simulink model "GMCLIB_Park_BAM_F32"  (Simulink 8.3)
settings: Solver=ode45  StartTime=0.0  StopTime=10.0  RelTol=1e-3
settings Model: Creator=RE004C  LastModifiedBy=B17364
settings OptimizationCC: ExpressionDepthLimit=2147483647
settings DebuggingCC: FcnCallInpInsideContextMsg=UseLocalSettings  StrictBusMsg=Warning
settings HardwareCC: ProdLargestAtomicInteger=Long  ProdLargestAtomicFloat=Double  ProdIntDivRoundTo=Zero  ProdEndianess=BigEndian  ProdHWDeviceType=Freescale->32-bit PowerPC

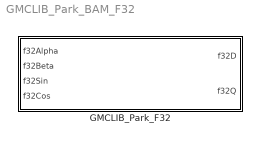
== system GMCLIB_Park_BAM_F32 ==
  GMCLIB_Park_F32 : Subsystem  mask(GMCLIB_Park_F32){}
      mask help: Bit accurate model of Park transformation 2ph stationary -> 2ph rotational.
      mask init:
      | pos = get_param(gcb, 'Position');width = pos(3) - pos(1); height = pos(4) - pos(2);tX=width/2;tY=height*0.9;
      mask Display: color('black');port_label('input',1,'f32Alpha');port_label('input',2,'f32Beta');port_label('input',3,'f32Sin');port_label('input',4,'f32Cos');port_label('output',1,'f32D');port_label('output',2,'f32Q');color('black');disp('GMCLIB_Park_F32');color('blue');text(tX,tY, 'BAM', 'horizontalAlignment', 'center');

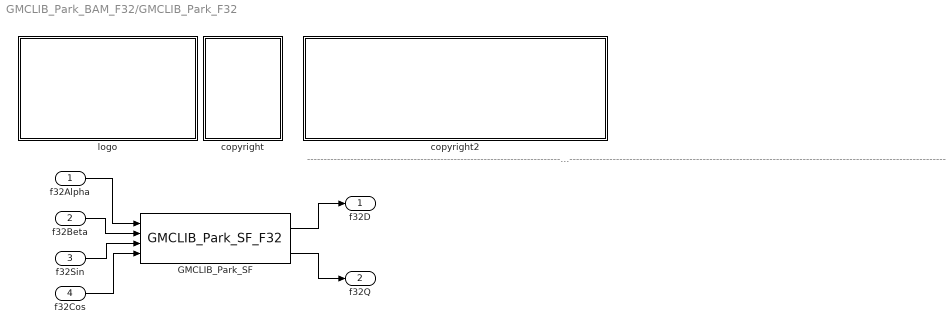
== system GMCLIB_Park_BAM_F32/GMCLIB_Park_F32 ==
  note: ---------------------------------------------------------------------------------------------------------------------------------------------------------------------------------------------------
  f32Alpha : Inport
  f32Beta : Inport  Port=2
  f32Sin : Inport  Port=3
  f32Cos : Inport  Port=4
  GMCLIB_Park_SF : S-Function  FunctionName=GMCLIB_Park_SF_F32  EnableBusSupport=off
  copyright : Subsystem
      mask Display:
      | text(10,90,'FILE:');text(10,75,'DESRIPTION:')
      | text(10,60,'COPYRIGHT:')
      | text(10,45,'VERSION:')
      | text(10,30,'DATE:')
  copyright2 : Subsystem
      mask Display:
      | text(10,90,'GMCLIB_Park_BAM_F32.mdl');text(10,75,'Park transformation.');text(10,60,'Freescale')
      | text(10,45,'0.1');text(10,30,'19-Sep-2011');
  logo : Subsystem
      mask Display: image(imread('logo.jpg'))
  f32D : Outport
  f32Q : Outport  Port=2
  wires:
  f32Alpha/1 -> GMCLIB_Park_SF/1
  f32Beta/1 -> GMCLIB_Park_SF/2
  f32Sin/1 -> GMCLIB_Park_SF/3
  f32Cos/1 -> GMCLIB_Park_SF/4
  GMCLIB_Park_SF/1 -> f32D/1
  GMCLIB_Park_SF/2 -> f32Q/1

== system GMCLIB_Park_BAM_F32/GMCLIB_Park_F32/copyright ==

== system GMCLIB_Park_BAM_F32/GMCLIB_Park_F32/copyright2 ==

== system GMCLIB_Park_BAM_F32/GMCLIB_Park_F32/logo ==
